simulink model "simple_walk_3d_robot"  (R2015a)
settings: Solver=FixedStepDiscrete  StartTime=0.0  StopTime=inf  FixedStep=sample_time  RelTol=1e-3
values from neighbouring files (symbols this model uses):
  sample_time = 1/sample_freq    (= 0.001)    [simulation_params.m]
settings Model: SimulationMode=external  CovSFcnEnable=off  Creator=wmartin  LastModifiedBy=robots
settings SolverCC: EnableConcurrentExecution=on
settings DataIOCC: LimitDataPoints=off  MaxDataPoints=1e7  SaveFormat=StructureWithTime  SignalLogging=off  DSMLogging=off
settings OptimizationCC: BlockReduction=off  OptimizeBlockIOStorage=off  BufferReuse=off  GlobalBufferReuse=off  ExpressionFolding=off  ExpressionDepthLimit=2147483647  LocalBlockOutputs=off  SimCompilerOptimization=on
settings DebuggingCC: UnderspecifiedInitializationDetection=Classic  MergeDetectMultiDrivingBlocksExec=none  SolverPrmCheckMsg=warning  StateNameClashWarn=warning
settings HardwareCC: ProdIntDivRoundTo=Zero  ProdEndianess=LittleEndian  ProdLongLongMode=on  ProdHWDeviceType=Generic->32-bit x86 compatible
settings ModelReferenceCC: UpdateModelReferenceTargets=IfOutOfDate  ModelReferenceNumInstancesAllowed=Single  ModelReferenceMinAlgLoopOccurrences=on
settings RTWCC: SystemTargetFile=slrt.tlc  TemplateMakefile=slrt_default_tmf  Description=Simulink Real-Time  RTWVerbose=off  RTWCompilerOptimization=on
settings CodeAppCC: MaxIdLength=256
settings SimulinkRealTimeCC: GeneratePreprocessorConditionals=Disable all  RL32LogBufSizeModifier=1e8

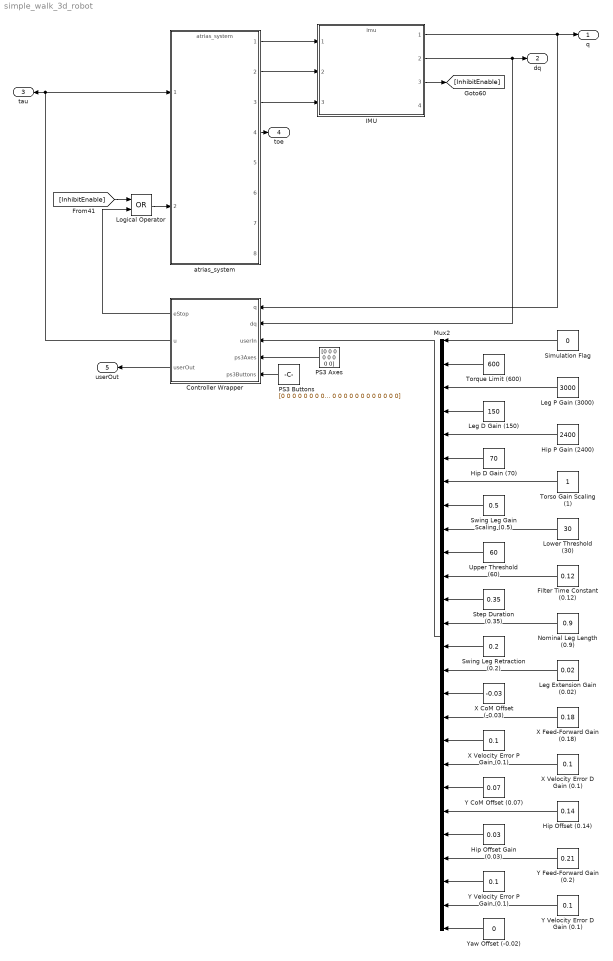
== system simple_walk_3d_robot ==
  Controller Wrapper : MATLAB Function  TreatAsAtomicUnit=on
  Filter Time Constant (0.12) : Constant  Value=0.12  SampleTime=sample_time
  Hip D Gain (70) : Constant  Value=70  SampleTime=sample_time
  Hip Offset (0.14) : Constant  Value=0.14  SampleTime=sample_time
  Hip Offset Gain (0.03) : Constant  Value=0.03  SampleTime=sample_time
  Hip P Gain (2400) : Constant  Value=2400  SampleTime=sample_time
  IMU : ModelReference  ModelNameDialog=imu  SimulationMode=Normal  ModelReferenceVersion=1.2451  CopyOfModelName=imu  DefaultDataLogging=on
  Leg D Gain (150) : Constant  Value=150  SampleTime=sample_time
  Leg Extension Gain (0.02) : Constant  Value=0.02  SampleTime=sample_time
  Leg P Gain (3000) : Constant  Value=3000  SampleTime=sample_time
  Logical Operator : Logic  Operator=OR  AllPortsSameDT=off  OutDataTypeStr=boolean
  Lower Threshold (30) : Constant  Value=30  SampleTime=sample_time
  Mux2 : Mux  Inputs=26
  Nominal Leg Length (0.9) : Constant  Value=0.9  SampleTime=sample_time
  PS3 Axes : Constant  Value=[0 0 0 0 0 0 0 0]
  PS3 Buttons : Constant  Value=[0 0 0 0 0 0 0 0 0 0 0 0 0 0 0 0 0 0 0 0]
  Simulation Flag : Constant  Value=0  SampleTime=sample_time
  Step Duration (0.35) : Constant  Value=0.35  SampleTime=sample_time
  Swing Leg Gain Scaling (0.5) : Constant  Value=0.5  SampleTime=sample_time
  Swing Leg Retraction (0.2) : Constant  Value=0.2  SampleTime=sample_time
  Torque Limit (600) : Constant  Value=600  SampleTime=sample_time
  Torso Gain Scaling (1) : Constant  SampleTime=sample_time
  Upper Threshold (60) : Constant  Value=60  SampleTime=sample_time
  X CoM Offset (-0.03) : Constant  Value=-0.03  SampleTime=sample_time
  X Feed-Forward Gain (0.18) : Constant  Value=0.18  SampleTime=sample_time
  X Velocity Error D Gain (0.1) : Constant  Value=0.1  SampleTime=sample_time
  X Velocity Error P Gain (0.1) : Constant  Value=0.1  SampleTime=sample_time
  Y CoM Offset (0.07) : Constant  Value=0.07  SampleTime=sample_time
  Y Feed-Forward Gain (0.2) : Constant  Value=0.21  SampleTime=sample_time
  Y Velocity Error D Gain (0.1) : Constant  Value=0.1  SampleTime=sample_time
  Y Velocity Error P Gain (0.1) : Constant  Value=0.1  SampleTime=sample_time
  Yaw Offset (-0.02) : Constant  Value=0  SampleTime=sample_time
  atrias_system : ModelReference  ModelNameDialog=atrias_system  SimulationMode=Normal  ModelReferenceVersion=1.2630  CopyOfModelName=atrias_system  DefaultDataLogging=on
  q : Outport
  dq : Outport  Port=2
  tau : Outport  Port=3
  toe : Outport  Port=4
  userOut : Outport  Port=5
  wires:
  Controller Wrapper/2(u) -> atrias_system/1, tau/1
  atrias_system/4 -> toe/1
  IMU/3 -> [InhibitEnable]
  Logical Operator/1 -> atrias_system/2
  [InhibitEnable] -> Logical Operator/1
  Controller Wrapper/1(eStop) -> Logical Operator/2
  IMU/1 -> Controller Wrapper/1(q), q/1
  IMU/2 -> Controller Wrapper/2(dq), dq/1
  atrias_system/1 -> IMU/1
  atrias_system/2 -> IMU/2
  atrias_system/3 -> IMU/3
  PS3 Axes/1 -> Controller Wrapper/4(ps3Axes)
  Controller Wrapper/3(userOut) -> userOut/1
  PS3 Buttons/1 -> Controller Wrapper/5(ps3Buttons)
  Mux2/1 -> Controller Wrapper/3(userIn)
  Torque Limit (600)/1 -> Mux2/2
  Leg P Gain (3000)/1 -> Mux2/3
  Leg D Gain (150)/1 -> Mux2/4
  Hip P Gain (2400)/1 -> Mux2/5
  Hip D Gain (70)/1 -> Mux2/6
  Simulation Flag/1 -> Mux2/1
  Torso Gain Scaling (1)/1 -> Mux2/7
  Swing Leg Gain Scaling (0.5)/1 -> Mux2/8
  Lower Threshold (30)/1 -> Mux2/9
  Upper Threshold (60)/1 -> Mux2/10
  Filter Time Constant (0.12)/1 -> Mux2/11
  Step Duration (0.35)/1 -> Mux2/12
  Nominal Leg Length (0.9)/1 -> Mux2/13
  Swing Leg Retraction (0.2)/1 -> Mux2/14
  Y Velocity Error D Gain (0.1)/1 -> Mux2/25
  Yaw Offset (-0.02)/1 -> Mux2/26
  Y Velocity Error P Gain (0.1)/1 -> Mux2/24
  Y Feed-Forward Gain (0.2)/1 -> Mux2/23
  Hip Offset Gain (0.03)/1 -> Mux2/22
  Hip Offset (0.14)/1 -> Mux2/21
  Y CoM Offset (0.07)/1 -> Mux2/20
  X Velocity Error D Gain (0.1)/1 -> Mux2/19
  X Velocity Error P Gain (0.1)/1 -> Mux2/18
  X Feed-Forward Gain (0.18)/1 -> Mux2/17
  X CoM Offset (-0.03)/1 -> Mux2/16
  Leg Extension Gain (0.02)/1 -> Mux2/15

== matlab function simple_walk_3d_robot/Controller Wrapper ==
  data: q input; dq input; userIn input; ps3Axes input; eStop output; u output; userOut output; ps3Buttons input
function [eStop, u, userOut] = wrapper(q, dq, userIn, ps3Axes, ps3Buttons)
%WRAPPER Controller wrapper.
%
% Notes:
% 	- State indexes (q and qdot)
%       (rBl rBm rAl rAm lBl lBm lAl lAm rHm lHm bR bY bP) 
%   - Input indexes (u)
%       (rB rA rH lB lA lH)
    
    % Actual controller function
    [eStop, u, userOut] = controller(q, dq, userIn, ps3Axes, ps3Buttons);
end % wrapper
